simulink model "ControladoresEjemplo"  (R2018b)
settings: Solver=VariableStepAuto  StartTime=0.0  StopTime=10.0  RelTol=1e-3
settings Model: Creator=jarico  LastModifiedBy=jarico

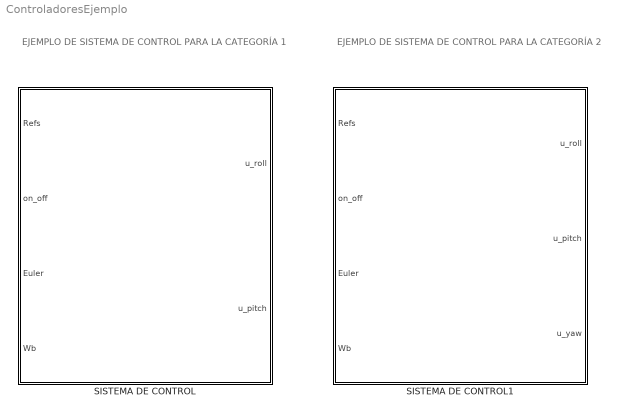
== system ControladoresEjemplo ==
  note: EJEMPLO DE SISTEMA DE CONTROL
      | PARA LA CATEGORÍA 1
  note: EJEMPLO DE SISTEMA DE CONTROL
      | PARA LA CATEGORÍA 2
  SISTEMA DE CONTROL : Subsystem
  SISTEMA DE CONTROL1 : Subsystem

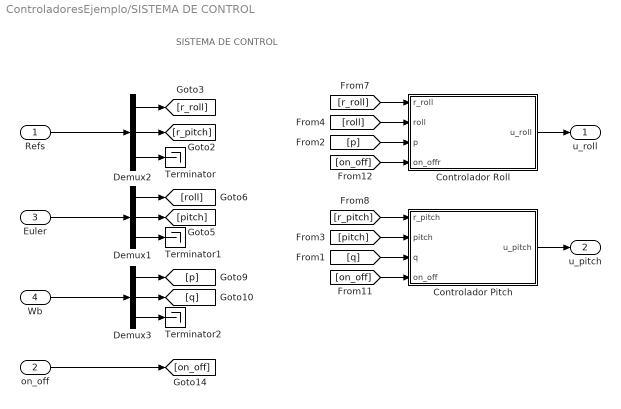
== system ControladoresEjemplo/SISTEMA DE CONTROL ==
  note: SISTEMA DE CONTROL
  Refs : Inport
  on_off : Inport  Port=2
  Euler : Inport  Port=3
  Wb : Inport  Port=4
  Controlador Pitch : Subsystem
  Controlador Roll : Subsystem
  Demux1 : Demux  Outputs=3
  Demux2 : Demux  Outputs=3
  Demux3 : Demux  Outputs=3
  Terminator : Terminator
  Terminator1 : Terminator
  Terminator2 : Terminator
  u_roll : Outport
  u_pitch : Outport  Port=2
  wires:
  Demux3/1 -> [p]
  Demux3/2 -> [q]
  Demux3/3 -> Terminator2/1
  Demux1/1 -> [roll]
  Demux1/2 -> [pitch]
  Demux1/3 -> Terminator1/1
  [p] -> Controlador Roll/3(p)
  [roll] -> Controlador Roll/2(roll)
  [r_roll] -> Controlador Roll/1(r_roll)
  Refs/1 -> Demux2/1
  Controlador Pitch/1(u_pitch) -> u_pitch/1
  Controlador Roll/1(u_roll) -> u_roll/1
  Demux2/1 -> [r_roll]
  Demux2/2 -> [r_pitch]
  Demux2/3 -> Terminator/1
  on_off/1 -> [on_off]
  [on_off] -> Controlador Roll/4(on_offr)
  [r_pitch] -> Controlador Pitch/1(r_pitch)
  [pitch] -> Controlador Pitch/2(pitch)
  [q] -> Controlador Pitch/3(q)
  [on_off] -> Controlador Pitch/4(on_off)
  Euler/1 -> Demux1/1
  Wb/1 -> Demux3/1

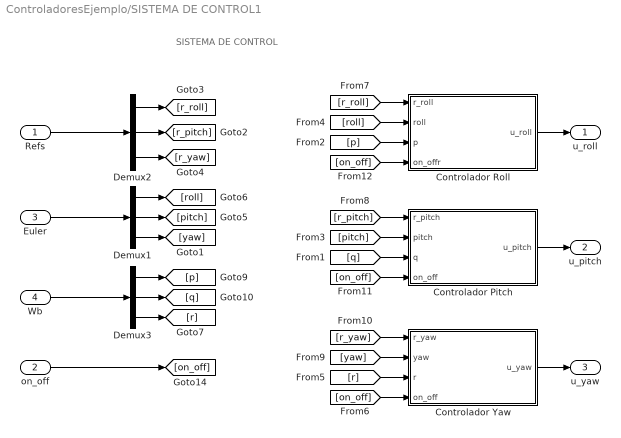
== system ControladoresEjemplo/SISTEMA DE CONTROL1 ==
  note: SISTEMA DE CONTROL
  Refs : Inport
  on_off : Inport  Port=2
  Euler : Inport  Port=3
  Wb : Inport  Port=4
  Controlador Pitch : Subsystem
  Controlador Roll : Subsystem
  Controlador Yaw : Subsystem
  Demux1 : Demux  Outputs=3
  Demux2 : Demux  Outputs=3
  Demux3 : Demux  Outputs=3
  u_roll : Outport
  u_pitch : Outport  Port=2
  u_yaw : Outport  Port=3
  wires:
  Demux3/1 -> [p]
  Demux3/2 -> [q]
  Demux3/3 -> [r]
  Demux1/1 -> [roll]
  Demux1/2 -> [pitch]
  Demux1/3 -> [yaw]
  [p] -> Controlador Roll/3(p)
  [roll] -> Controlador Roll/2(roll)
  [r_roll] -> Controlador Roll/1(r_roll)
  Refs/1 -> Demux2/1
  Controlador Pitch/1(u_pitch) -> u_pitch/1
  Controlador Roll/1(u_roll) -> u_roll/1
  Demux2/1 -> [r_roll]
  Demux2/2 -> [r_pitch]
  Demux2/3 -> [r_yaw]
  on_off/1 -> [on_off]
  [on_off] -> Controlador Roll/4(on_offr)
  [r_pitch] -> Controlador Pitch/1(r_pitch)
  [pitch] -> Controlador Pitch/2(pitch)
  [q] -> Controlador Pitch/3(q)
  [on_off] -> Controlador Pitch/4(on_off)
  Euler/1 -> Demux1/1
  Wb/1 -> Demux3/1
  Controlador Yaw/1(u_yaw) -> u_yaw/1
  [on_off] -> Controlador Yaw/4(on_off)
  [r] -> Controlador Yaw/3(r)
  [yaw] -> Controlador Yaw/2(yaw)
  [r_yaw] -> Controlador Yaw/1(r_yaw)

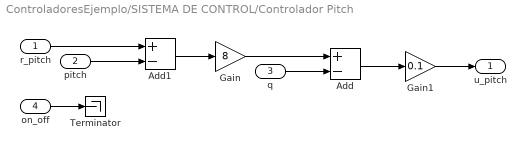
== system ControladoresEjemplo/SISTEMA DE CONTROL/Controlador Pitch ==
  r_pitch : Inport
  pitch : Inport  Port=2
  q : Inport  Port=3
  on_off : Inport  Port=4
  Add : Sum  Inputs=+-
  Add1 : Sum  Inputs=+-
  Gain : Gain  Gain=8
  Gain1 : Gain  Gain=0.1
  Terminator : Terminator
  u_pitch : Outport
  wires:
  Gain1/1 -> u_pitch/1
  Add1/1 -> Gain/1
  on_off/1 -> Terminator/1
  pitch/1 -> Add1/2
  q/1 -> Add/2
  Gain/1 -> Add/1
  Add/1 -> Gain1/1
  r_pitch/1 -> Add1/1

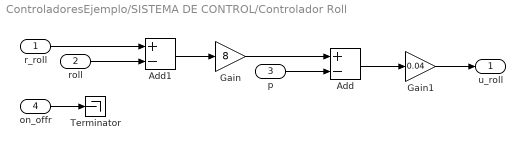
== system ControladoresEjemplo/SISTEMA DE CONTROL/Controlador Roll ==
  r_roll : Inport
  roll : Inport  Port=2
  p : Inport  Port=3
  on_offr : Inport  Port=4
  Add : Sum  Inputs=+-
  Add1 : Sum  Inputs=+-
  Gain : Gain  Gain=8
  Gain1 : Gain  Gain=0.04
  Terminator : Terminator
  u_roll : Outport
  wires:
  r_roll/1 -> Add1/1
  Add/1 -> Gain1/1
  Gain/1 -> Add/1
  p/1 -> Add/2
  roll/1 -> Add1/2
  on_offr/1 -> Terminator/1
  Add1/1 -> Gain/1
  Gain1/1 -> u_roll/1

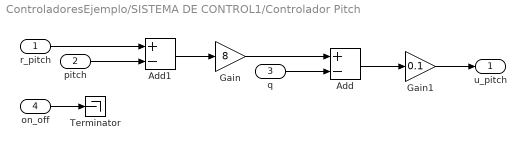
== system ControladoresEjemplo/SISTEMA DE CONTROL1/Controlador Pitch ==
  r_pitch : Inport
  pitch : Inport  Port=2
  q : Inport  Port=3
  on_off : Inport  Port=4
  Add : Sum  Inputs=+-
  Add1 : Sum  Inputs=+-
  Gain : Gain  Gain=8
  Gain1 : Gain  Gain=0.1
  Terminator : Terminator
  u_pitch : Outport
  wires:
  Gain1/1 -> u_pitch/1
  Add1/1 -> Gain/1
  on_off/1 -> Terminator/1
  pitch/1 -> Add1/2
  q/1 -> Add/2
  Gain/1 -> Add/1
  Add/1 -> Gain1/1
  r_pitch/1 -> Add1/1

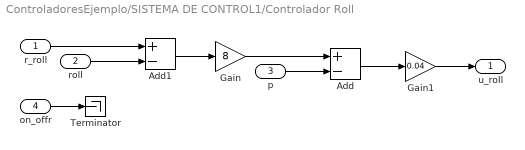
== system ControladoresEjemplo/SISTEMA DE CONTROL1/Controlador Roll ==
  r_roll : Inport
  roll : Inport  Port=2
  p : Inport  Port=3
  on_offr : Inport  Port=4
  Add : Sum  Inputs=+-
  Add1 : Sum  Inputs=+-
  Gain : Gain  Gain=8
  Gain1 : Gain  Gain=0.04
  Terminator : Terminator
  u_roll : Outport
  wires:
  r_roll/1 -> Add1/1
  Add/1 -> Gain1/1
  Gain/1 -> Add/1
  p/1 -> Add/2
  roll/1 -> Add1/2
  on_offr/1 -> Terminator/1
  Add1/1 -> Gain/1
  Gain1/1 -> u_roll/1

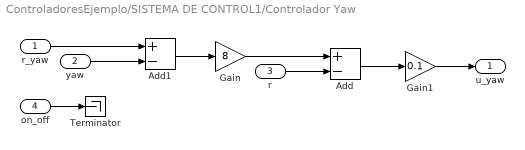
== system ControladoresEjemplo/SISTEMA DE CONTROL1/Controlador Yaw ==
  r_yaw : Inport
  yaw : Inport  Port=2
  r : Inport  Port=3
  on_off : Inport  Port=4
  Add : Sum  Inputs=+-
  Add1 : Sum  Inputs=+-
  Gain : Gain  Gain=8
  Gain1 : Gain  Gain=0.1
  Terminator : Terminator
  u_yaw : Outport
  wires:
  r_yaw/1 -> Add1/1
  Add/1 -> Gain1/1
  Gain/1 -> Add/1
  r/1 -> Add/2
  yaw/1 -> Add1/2
  on_off/1 -> Terminator/1
  Add1/1 -> Gain/1
  Gain1/1 -> u_yaw/1
